simulink model "SampleForC"  (R2020a)
settings: Solver=FixedStepAuto  StartTime=0.0  StopTime=inf  RelTol=1e-3  EnableMultiTasking=on
settings Model: Creator=eisuk  LastModifiedBy=eisuk
settings SolverCC: PositivePriorityOrder=on
settings OptimizationCC: EnhancedBackFolding=on  PassReuseOutputArgsAs=Individual arguments  ZeroExternalMemoryAtStartup=off  ZeroInternalMemoryAtStartup=off  MaxStackSize=64  OptimizeBlockOrder=speed  DifferentSizesBufferReuse=on  OptimizationCustomize=off  EfficientTunableParamExpr=on
settings DebuggingCC: ParameterTunabilityLossMsg=error
settings HardwareCC: ProdBitPerPointer=32  ProdBitPerSizeT=32  ProdBitPerPtrDiffT=32  ProdLargestAtomicInteger=Long  ProdLargestAtomicFloat=Double  ProdWordSize=32  ProdLongLongMode=on  ProdHWDeviceType=ARM Compatible->ARM Cortex
settings RTWCC: SystemTargetFile=ert.tlc  HardwareBoard=Raspberry Pi  TemplateMakefile=ert_default_tmf  Toolchain=GNU GCC Raspberry Pi  BuildConfiguration=Faster Runs
settings CodeAppCC: ForceParamTrailComments=on  IgnoreCustomStorageClasses=off  OperatorAnnotations=on  SimulinkDataObjDesc=on  SFDataObjDesc=on  InsertBlockDesc=on
settings ERTTargetCC: SupportVariableSizeSignals=on

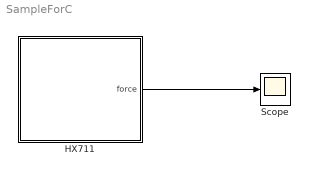
== system SampleForC ==
  HX711 : Subsystem  mask{doutPin=17, sckPin=27, rate=10 SPS, offset=0, scale=1}
      mask prompts: doutPin "DOUT Pin Number:"; sckPin "PD_SCK Pin Number:"; rate "Data rate:"; offset "Offset :"; scale "Scale :"
      mask init:
      | switch rate
      |     case 1
      |         sampleTime = 1/10;
      |     case 2
      |         sampleTime = 1/80;
      | end
      mask TypeOptions doutPin: MATLAB System/doutPin
      mask TypeOptions sckPin: MATLAB System/sckPin
      mask TypeOptions rate: 10 SPS | 80 SPS
      mask TypeOptions offset: getPhysicalQuantity/offset
      mask TypeOptions scale: getPhysicalQuantity/scale
      mask Display:
      | h = get_param(gcb, 'MaskValues');
      | text(0.5, 0.5, 'HX711 A/D Converter', 'horizontalAlignment', 'center');
      | text(0.2, 0.2, [' DOUT Pin: ', h{1}, ...
      |                 '\n PD_SCK Pin: ', h{2},...
      |                 '\n Data Rate: ', h{3}],...
      |                 'horizontalAlignment', 'left');
      | color('blue');
      | text(0.90, 0.90, 'RASPBERRYPI', 'horizontalAlignment', 'right');
      | color('black');
  Scope : Scope
  wires:
  HX711/1(force) -> Scope/1

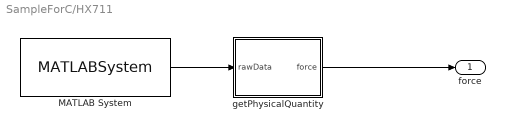
== system SampleForC/HX711 ==
  MATLAB System : MATLABSystem  System=HX711Driver  doutPin=doutPin  sckPin=sckPin  SampleTime=sampleTime
      mask Type: HX711Driver
      mask Display:
      | disp('HX711Driver');
      | port_label('output',1,'rawData');
  getPhysicalQuantity : Subsystem  mask{offset=offset, scale=scale}
      mask prompts: offset "Offset :"; scale "Scale :"
  force : Outport
  wires:
  getPhysicalQuantity/1(force) -> force/1
  MATLAB System/1 -> getPhysicalQuantity/1(rawData)

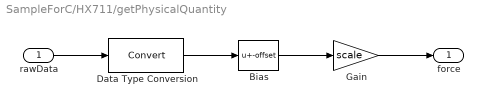
== system SampleForC/HX711/getPhysicalQuantity ==
  rawData : Inport
  Bias : Bias  Bias=-offset
  Data Type Conversion : DataTypeConversion
  Gain : Gain  Gain=scale
  force : Outport
  wires:
  Gain/1 -> force/1
  Data Type Conversion/1 -> Bias/1
  rawData/1 -> Data Type Conversion/1
  Bias/1 -> Gain/1
